simulink model "udp_sender_18b"  (R2018b)
settings: Solver=ode2  StartTime=0.0  StopTime=100  FixedStep=1/30  RelTol=1e-3
undefined symbols (not defined in the file or in its folder): aircraft
libraries: qt_opengl_visualization_lib x1, aerolibanimutils x1
settings Model: Creator=akuzolap  LastModifiedBy=fabian
settings DataIOCC: ReturnWorkspaceOutputs=on

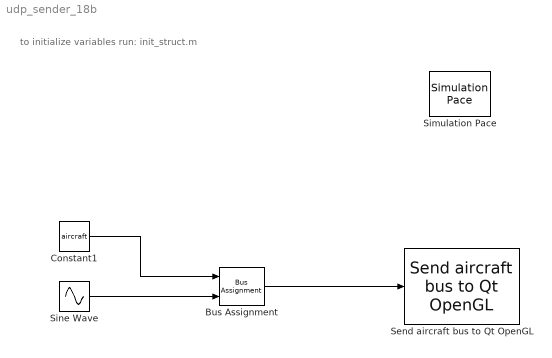
== system udp_sender_18b ==
  note: to initialize variables run: init_struct.m
  Bus Assignment : BusAssignment  AssignedSignals=wing.geometry.vortex.z
  Constant1 : Constant  Value=aircraft  OutDataTypeStr=Bus: aircraftBus
  Send aircraft bus to Qt OpenGL : qt_opengl_visualization_lib/Send aircraft bus to Qt OpenGL  sample_time=1/30  ip_address='192.168.11.5'  ip_port=4321  aircraftDouble=aircraftDoubleArray  aircraftIdx=aircraftDoubleIdx
  Simulation Pace : aerolibanimutils/Simulation Pace  SimulationPace=1  SleepMode=Auto  OutputPaceError=off  SampleTime=1/30
  Sine Wave : Sin  Amplitude=0.07*rand(5,1)  Frequency=5*rand(5,1)  SampleTime=0
  wires:
  Constant1/1 -> Bus Assignment/1
  Sine Wave/1 -> Bus Assignment/2
  Bus Assignment/1 -> Send aircraft bus to Qt OpenGL/1
